simulink model "ecg_modelo_hil"  (Simulink 8.1)
settings: Solver=ode5  StartTime=0.0  StopTime=inf  RelTol=1e-3
undefined symbols (not defined in the file): National_Instruments, PCI, Ts
libraries: rtwinlib x1, commnoisgen2 x1
Description:
  | Real-Time Signal Generator
  | 
  | This demonstration shows how to produce an analog output signal using
  | Real-Time Windows Target. Because analog output typically requires
  | less configuration and is easier to connect than analog input, this demo
  | is a good start to your experiments with data acquisition boards. You can
  | verify the presence of the generated signal e.g. by connecting an
  | oscilloscope to the analog output pins of your data acquisition board.
  | 
  | How to run this demo:
  | 
  |   1. Open the Analog Output block and select your data acquisition board.
  |       If there's no board installed, install it using the Install new board button.
  |   2. Build the model using Tools -> Code Generation -> Build Model.
  |   3. Connect to the real-time code using Simulation -> Connect to target.
  |   4. Start the real-time execution using Simulation -> Start real-time code.
  | 
  | Note:
  | To run this demo, you must have a data acquisition board plugged into your computer.
settings Model: Creator=The MathWorks Inc.  LastModifiedBy=rafa  SimulationMode=external  ExtModeTrigType=signal  ExtModeTrigLevel=0.500000
settings DataIOCC: SignalLoggingName=logsOut
settings OptimizationCC: InitFltsAndDblsToZero=on  EfficientMapNaN2IntZero=off
settings DebuggingCC: SignalResolutionControl=TryResolveAllWithWarning  SolverPrmCheckMsg=none  StrictBusMsg=Warning
settings HardwareCC: ProdIntDivRoundTo=Zero  ProdEndianess=LittleEndian  ProdHWDeviceType=32-bit Real-Time Windows Target
settings RTWCC: SystemTargetFile=rtwin.tlc  TemplateMakefile=rtwin.tmf  Description=Real-Time Windows Target  ProcessScript=rtwin_make_rtw_hook
settings TargetCC: TargetLibSuffix=_rtwin.lib  TargetPreCompLibLocation=C:\Program Files\MATLAB\R2011a\toolbox\rtw\targets\rtwin\lib\win32  CodeReplacementLibrary=ANSI_C  IsPILTarget=off  EnableShiftOperators=on
settings CustomProperty: DataType=string

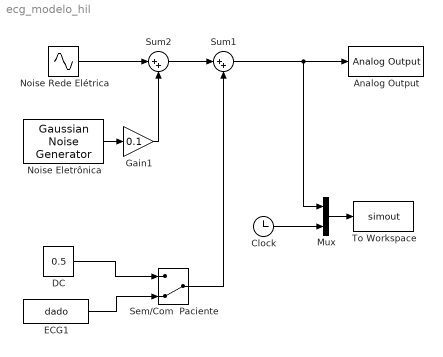
== system ecg_modelo_hil ==
  Analog Output : rtwinlib/Analog Output  SampleTime=1e-3  DrvName=National_Instruments/PCI-6251  DrvAddress=4294967295  DrvOptions=[0 0 0 0 0]  Channels=1:2  RangeMode=1  VoltRange=1  InitialValue=[]  FinalValue=[]
      settings: AttributesFormatString=National Instruments\nPCI-6251 [auto]
  Clock : Clock
  DC : Constant  Value=0.5  SampleTime=Ts
  ECG1 : FromWorkspace  VariableName=dado  SampleTime=Ts  Interpolate=off  OutputAfterFinalValue=Cyclic repetition
  Gain1 : Gain  Gain=0.1  SampleTime=Ts
  Mux : Mux  Inputs=2
  Noise Eletrônica : commnoisgen2/Gaussian Noise Generator  m=0  d=1  s=41  Ts=Ts  frameBased=off  sampPerFrame=1  orient=off  outDataType=double
  Noise Rede Elétrica : Sin  Amplitude=0.6  Frequency=60*2*pi  Samples=60  SampleTime=Ts
  Sem/Com  Paciente : ManualSwitch  CurrentSetting=0
  Sum1 : Sum  Inputs=|++  SampleTime=Ts
  Sum2 : Sum  Inputs=|++  SampleTime=Ts
  To Workspace : ToWorkspace  VariableName=simout  SampleTime=-1
  wires:
  Sum1/1 -> Analog Output/1, Mux/1
  Mux/1 -> To Workspace/1
  Clock/1 -> Mux/2
  Noise Rede Elétrica/1 -> Sum2/1
  Sum2/1 -> Sum1/1
  Noise Eletrônica/1 -> Gain1/1
  Gain1/1 -> Sum2/2
  ECG1/1 -> Sem/Com  Paciente/2
  DC/1 -> Sem/Com  Paciente/1
  Sem/Com  Paciente/1 -> Sum1/2
